simulink model "untitled1"  (R2021b)
settings: Solver=VariableStepAuto  StartTime=0.0  StopTime=106.1385  RelTol=1e-3
values from neighbouring files (symbols this model uses):
  refPosesT = [timeVector, smoothRefPoses(:,3)]    [Copy_2_of_lidar_script.m]    (also in Copy_of_lidar_script.m; LiDARDrew.m = yawData.refPosesT; lidar_script.m = yawData.refPosesT)
  refPosesX = [timeVector, smoothRefPoses(:,1)]    [Copy_2_of_lidar_script.m]    (also in Copy_of_lidar_script.m; LiDARDrew.m = xData.refPosesX; lidar_script.m = xData.refPosesX)
  refPosesY = [timeVector, smoothRefPoses(:,2)]    [Copy_2_of_lidar_script.m]    (also in Copy_of_lidar_script.m; LiDARDrew.m = yData.refPosesY; lidar_script.m = yData.refPosesY)
libraries: sim3dphyssensorlib x1, sim3dlib x1, sim3dautolib x1
settings Model: Creator=Obama  LastModifiedBy=Obama

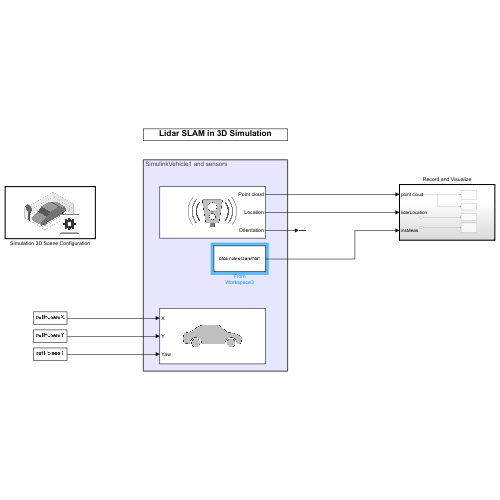
[thumbnail: Simulink's stored preview of the top-level diagram]
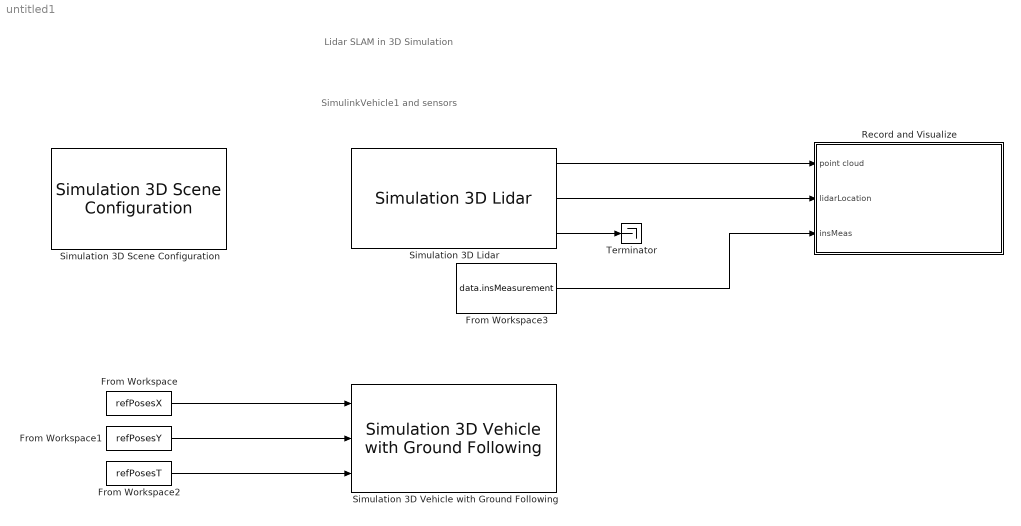
== system untitled1 ==
  note: Lidar SLAM in 3D Simulation
  note: SimulinkVehicle1 and sensors
  From Workspace : FromWorkspace  VariableName=refPosesX  OutputAfterFinalValue=Holding final value
  From Workspace1 : FromWorkspace  VariableName=refPosesY  OutputAfterFinalValue=Holding final value
  From Workspace2 : FromWorkspace  VariableName=refPosesT  Interpolate=off  OutputAfterFinalValue=Holding final value
  From Workspace3 : FromWorkspace  VariableName=data.insMeasurement  SampleTime=0.1  Interpolate=off  OutputAfterFinalValue=Holding final value
  Record and Visualize : Subsystem  TreatAsAtomicUnit=on
  Simulation 3D Lidar : sim3dphyssensorlib/Simulation 3D Lidar  sensorTag=Sim3dSensor1  sensorId=1  sensorName=Sim3dSensor1  vehTagList={'Scene Origin'}  vehTag=Scene Origin  mountLoc=Origin  offsetFlag=off  tmountOffset=[0, 0, 0]  rmountOffset=[0, 0, 0]  DetectionRange=90  RangeResolution=0.002  VerticalFOV=40  VerticalResolution=1.25  HorizontalFOV=360  HorizontalResolution=0.332409972299169  DistanceOutportEnabled=off  TransformOutportEnabled=on  SampleTime=0.1  mountPoint=[0 0 0]  mountOrientation=[0 0 0]  aMode=3  ID=1
      settings: SourceProductBaseCode=AE,DR,UV,VE
  Simulation 3D Scene Configuration : sim3dlib/Simulation 3D Scene Configuration  Priority=0  ProjectFormat_internal=Default Scenes  ProjectFormat=Default Scenes  SceneDesc=US city block  ProjectName=C:\Program Files\MATLAB\R2021b\toolbox\shared\sim3d_projects\automotive_project\UE4\WindowsNoEditor\VehicleSimulation.exe  ScenePath=/Game/Maps/HwStrght  vehTagList={'Scene Origin'}  vehTag=Scene Origin  OpVisEn=off  Ts=0.1  EnableWindow=on  EnableWeather=off  SunAltitude=40.0  SunAzimuth=90  clouds=10  wind=1  fog=0  rain=0  sensorTag=MainCamera1  sensorId=1  sensorName=MainCamera1  mountLoc=Origin  offsetFlag=off  tmountOffset=[0, 0, 0]  rmountOffset=[0, 0, 0]  HorizontalResolution=1280  VerticalResolution=720  HorizontalFOV=60  mountPoint=[0 0 0]  mountOrientation=[0 0 0]  aMode=3  ID=1
      settings: SourceProductBaseCode=AE,DR,UV,VE
  Simulation 3D Vehicle with Ground Following : sim3dautolib/Simulation 3D Vehicle with Ground Following  Priority=-1  PassVehMesh=Hatchback  PassVehMesh_Internal=Hatchback  MeshPath=/MathWorksSimulation/Vehicles/Muscle/Meshes/SK_MuscleCar.SK_MuscleCar  TrackWidth=1.9  WheelBase=3  WheelRadius=0.35  VehColor=Red  VehColor_Internal=Red  InitialPos=[refPosesX(1,2), refPosesY(1,2), 0]  InitialRot=[0, 0, refPosesT(1,2)]  ActorName=SimulinkVehicle1  SampleTime=-1  ActorType=SimulinkVehicle  ID=1  aMode=3  ActorTag=SimulinkVehicle1  CoordinateScheme=ISO  VehLightsControl=off  HeadlightColor=[ 1, 1, 1 ]  HighBeamIntensity=100000  LowBeamIntensity=60000  HighBeamConeAngle=70  LowBeamConeAngle=70  LeftHeadlightOrientation=[ 0, 0 ]  RightHeadlightOrientation=[ 0, 0 ]  BrakelightIntensity=500  ReverselightIntensity=500  SignallightIntensity=500  SignallightPeriod=1  SignalPulseWidth=50  TransformOutportEnabled=off
      settings: SourceProductBaseCode=AE,DR,UV,VE
  Terminator : Terminator
  wires:
  Simulation 3D Lidar/3 -> Terminator/1
  From Workspace2/1 -> Simulation 3D Vehicle with Ground Following/3
  From Workspace3/1 -> Record and Visualize/3(insMeas)
  From Workspace/1 -> Simulation 3D Vehicle with Ground Following/1
  Simulation 3D Lidar/2 -> Record and Visualize/2(lidarLocation)
  Simulation 3D Lidar/1 -> Record and Visualize/1(point cloud)
  From Workspace1/1 -> Simulation 3D Vehicle with Ground Following/2

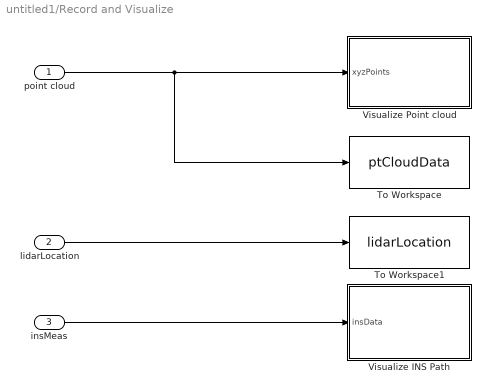
== system untitled1/Record and Visualize ==
  point cloud : Inport
  lidarLocation : Inport  Port=2
  insMeas : Inport  Port=3
  To Workspace : ToWorkspace  VariableName=ptCloudData  SaveFormat=Structure With Time  SampleTime=-1
  To Workspace1 : ToWorkspace  VariableName=lidarLocation  SaveFormat=Structure With Time  SampleTime=-1
  Visualize INS Path : MATLAB Function  StopFcn=|  TreatAsAtomicUnit=on
      | playerFigure = findall(groot,'type','figure','name','INS Sensor Display');
      | 
      | if ~isempty(playerFigure)
      |     playerFigure = playerFigure(end);
      |     if isvalid(playerFigure)
      |         close(playerFigure);
      |     end
      | end
  Visualize Point cloud : MATLAB Function  StopFcn=|  TreatAsAtomicUnit=on
      | playerFigure = findall(groot,'type','figure','name','Point Cloud Player');
      | 
      | if ~isempty(playerFigure)
      |     playerFigure = playerFigure(end);
      |     if isvalid(playerFigure)
      |         close(playerFigure);
      |     end
      | end
  wires:
  point cloud/1 -> To Workspace/1, Visualize Point cloud/1(xyzPoints)
  insMeas/1 -> Visualize INS Path/1(insData)
  lidarLocation/1 -> To Workspace1/1

== matlab function untitled1/Record and Visualize/Visualize INS Path ==
  data: insData input
function visualizeINSPath(insData)
%visualizeINSPath Visualize INS path on scene image
%   helperPlotPath plots the path specified by x,y waypoint on the current
%   scene.

% Copyright 2019 The MathWorks, Inc.

coder.extrinsic('helperShowSceneImage', 'figure', 'title', 'movegui', ...
    'isvalid', 'images.roi.Polyline', 'helperUpdatePolyline', 'xlim', 'ylim');

persistent hFig hPoly;

x = insData(1);
y = insData(2);

bufferZone = [30 30];

if isempty(hFig)
    % Query the model to find the scene selection
    sceneName = 'USCityBlock';
    
    % Create a figure and display the scene on it
    hFig = figure('Name', 'INS Sensor Display');
    helperShowSceneImage(sceneName);
    title('INS Sensor Display');
    
    % Move figure to right of screen
    movegui(hFig, 'east')
    
    % Display the path
    hold on
    hPoly = images.roi.Polyline('Parent', gca, 'Position', [x y], 'InteractionsAllowed', 'none');
end

if isvalid(hFig)
    % Update the path with the new point
    helperUpdatePolyline(hPoly, x, y);
    
    xlims = x + bufferZone(1)*[-1 1];
    ylims = y + bufferZone(2)*[-1 1];
    xlim(xlims);
    ylim(ylims);
end
end

== matlab function untitled1/Record and Visualize/Visualize Point cloud ==
  data: xyzPoints input
function VisualizePointCloud(xyzPoints)
%VisualizePointCloud Display point cloud

coder.extrinsic('isOpen', 'pcplayer')

persistent player;

if isempty(player)
    % Configure axes limits
    xlimits = [-90 90];
    ylimits = [-90 90];
    zlimits = [ -5 40];
    
    % Create a streaming Lidar viewer
    player = pcplayer(xlimits, ylimits, zlimits);
end

if ~isempty(player) && isOpen(player)
    view(player, xyzPoints);
end
